simulink model "TP_4"  (R2022a)
settings: Solver=VariableStepAuto  StartTime=0.0  StopTime=10.0  RelTol=1e-3
undefined symbols (not defined in the file): g, l
settings Model: Creator=acanon  LastModifiedBy=acanon

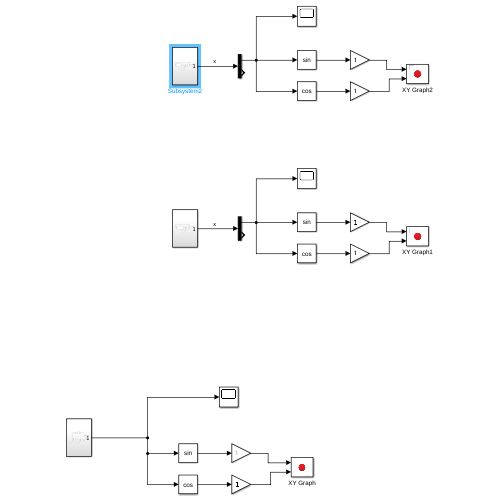
[thumbnail: Simulink's stored preview of the top-level diagram]
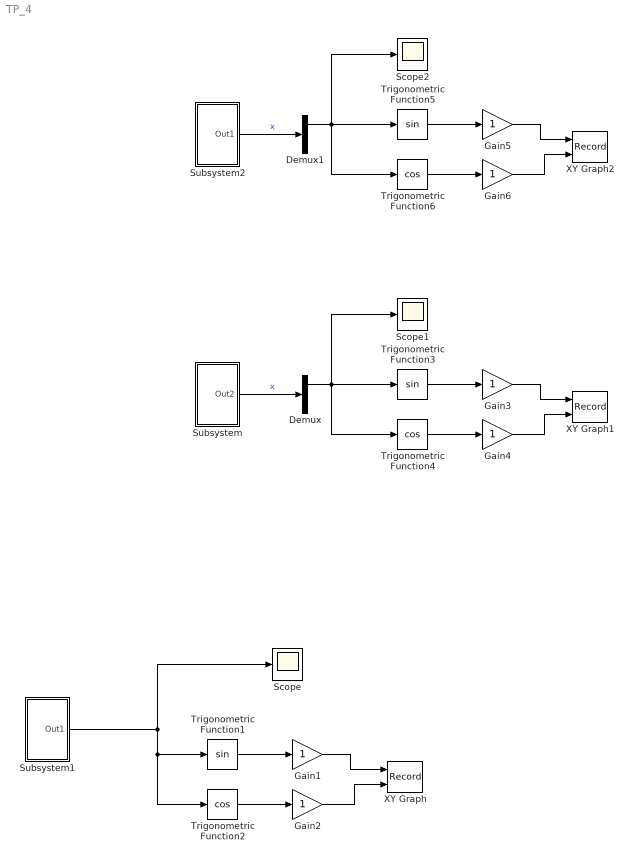
== system TP_4 ==
  Demux : Demux  Outputs=2
  Demux1 : Demux  Outputs=2
  Gain{1..6} (6 alike) : Gain
  Scope : Scope
  Scope1 : Scope
  Scope2 : Scope
  Subsystem : Subsystem
  Subsystem1 : Subsystem
  Subsystem2 : Subsystem
  Trigonometric Function1 : Trigonometry
  Trigonometric Function2 : Trigonometry  Operator=cos
  Trigonometric Function3 : Trigonometry
  Trigonometric Function4 : Trigonometry  Operator=cos
  Trigonometric Function5 : Trigonometry
  Trigonometric Function6 : Trigonometry  Operator=cos
  XY Graph : Record  FileSettingsInternal="{\"entries\":[{\"content\":{\"excelSettings\":{\"content\":{},\"type\":\"Streamout.ExcelSettings\"}},\"type\":\"Streamout.FileSettingStorage\",\"uuid\":\"6b5f49a7-b3b1-4d7e-bc90-530d4034afb4\"}],\"packageUris\":[\"http://schema.mathworks.com/mf0/streamout_blocks/R2020a\"],\"version\":\"1.0\"}"  Layout=[1 1]  SignalsInternal="{\"entries\":[{\"content\":{\"signals\":[{\"content\":{\"blockPath\":[\"TP_4/XY Graph\"],\"channel\":[],\"dimensions\":[1],\"domain\":\"TP_4/XY Graph\",\"lineColor\":\"#a2142f\",\"plots\":[1],\"port\":1,\"sid\":[\"\"],\"signalID\":770,\"signalName\":\"Gain1\"},\"type\":\"RecordBlkView.Signal\",\"uuid\":\"252f4a16-2fdb-4508-836e-7d7f95c59b1a\"},{\"content\":{\"blockPath\":[\"TP_4/XY Graph\"],\"channel\":[],\"dimensions\":[1],\"domain\":\"TP_4/XY Graph\",\"lineColor\":\"#139fff\",\"plots\":[1],\"port\":2,\"sid\":[\"\"],\"signalID\":774,\"signalName\":\"Gain2\"},\"type\":\"RecordBlkView.Signal\",\"uuid\":\"1550168d-e5f5-498f-8827-b1f3ffe8fbd9\"}]},\"type\":\"RecordBlkView.InputSignals\",\"uuid\":\"ba0f4b2c-9202-4a03-ae75-802def453182\"}],\"packageUris\":[\"http://schema.mathworks.com/mf0/streamout_blocks/R2020a\"],\"version\":\"1.0\"}"  VisualizationBindings="{\"xyplotplugin\":{\"info\":[{\"series\":[{\"bindingParametersList\":[{\"parameter\":\"X-Axis\",\"signalID\":770,\"signalName\":\"Gain1\"},{\"parameter\":\"Y-Axis\",\"signalID\":774,\"signalName\":\"Gain2\"}],\"seriesID\":7779}],\"subplotID\":1}]}}"  CompatibilityTag=XY
  XY Graph1 : Record  FileSettingsInternal="{\"entries\":[{\"content\":{\"excelSettings\":{\"content\":{},\"type\":\"Streamout.ExcelSettings\"}},\"type\":\"Streamout.FileSettingStorage\",\"uuid\":\"647a4500-99ce-4aa8-8361-fcd857458ba3\"}],\"packageUris\":[\"http://schema.mathworks.com/mf0/streamout_blocks/R2020a\"],\"version\":\"1.0\"}"  Layout=[1 1]  SignalsInternal="{\"entries\":[{\"content\":{\"signals\":[{\"content\":{\"blockPath\":[\"TP_4/XY Graph1\"],\"channel\":[],\"dimensions\":[1],\"domain\":\"TP_4/XY Graph1\",\"lineColor\":\"#a2142f\",\"plots\":[1],\"port\":1,\"sid\":[\"\"],\"signalID\":754,\"signalName\":\"Gain3\"},\"type\":\"RecordBlkView.Signal\",\"uuid\":\"8e395301-b303-424e-a96f-b943253f827c\"},{\"content\":{\"blockPath\":[\"TP_4/XY Graph1\"],\"channel\":[],\"dimensions\":[1],\"domain\":\"TP_4/XY Graph1\",\"lineColor\":\"#139fff\",\"plots\":[1],\"port\":2,\"sid\":[\"\"],\"signalID\":758,\"signalName\":\"Gain4\"},\"type\":\"RecordBlkView.Signal\",\"uuid\":\"861f5d7e-9fe7-4d07-8f40-ba319954fb9d\"}]},\"type\":\"RecordBlkView.InputSignals\",\"uuid\":\"dfbe973e-b0a0-4eca-b465-339f94536037\"}],\"packageUris\":[\"http://schema.mathworks.com/mf0/streamout_blocks/R2020a\"],\"version\":\"1.0\"}"  VisualizationBindings="{\"xyplotplugin\":{\"info\":[{\"series\":[{\"bindingParametersList\":[{\"parameter\":\"X-Axis\",\"signalID\":754,\"signalName\":\"Gain3\"},{\"parameter\":\"Y-Axis\",\"signalID\":758,\"signalName\":\"Gain4\"}],\"seriesID\":52056}],\"subplotID\":1}]}}"  CompatibilityTag=XY
  XY Graph2 : Record  FileSettingsInternal="{\"entries\":[{\"content\":{\"excelSettings\":{\"content\":{},\"type\":\"Streamout.ExcelSettings\"}},\"type\":\"Streamout.FileSettingStorage\",\"uuid\":\"91d296fc-894f-4125-a729-7558be06892a\"}],\"packageUris\":[\"http://schema.mathworks.com/mf0/streamout_blocks/R2020a\"],\"version\":\"1.0\"}"  Layout=[1 1]  SignalsInternal="{\"entries\":[{\"content\":{\"signals\":[{\"content\":{\"blockPath\":[\"TP_4/XY Graph2\"],\"channel\":[],\"dimensions\":[1,1],\"domain\":\"TP_4/XY Graph2\",\"lineColor\":\"#a2142f\",\"plots\":[1],\"port\":1,\"sid\":[\"\"],\"signalID\":762,\"signalName\":\"Gain5\"},\"type\":\"RecordBlkView.Signal\",\"uuid\":\"373c4582-ecbd-4420-a1ec-272adeca90e9\"},{\"content\":{\"blockPath\":[\"TP_4/XY Graph2\"],\"channel\":[],\"dimensions\":[1,1],\"domain\":\"TP_4/XY Graph2\",\"lineColor\":\"#139fff\",\"plots\":[1],\"port\":2,\"sid\":[\"\"],\"signalID\":766,\"signalName\":\"Gain6\"},\"type\":\"RecordBlkView.Signal\",\"uuid\":\"e2adde95-3a69-431b-804e-fdc9e32eb17f\"}]},\"type\":\"RecordBlkView.InputSignals\",\"uuid\":\"6b5ed82e-5b03-46e4-8a06-dd9cee375b8d\"}],\"packageUris\":[\"http://schema.mathworks.com/mf0/streamout_blocks/R2020a\"],\"version\":\"1.0\"}"  VisualizationBindings="{\"xyplotplugin\":{\"info\":[{\"series\":[{\"bindingParametersList\":[{\"parameter\":\"X-Axis\",\"signalID\":762,\"signalName\":\"Gain5\"},{\"parameter\":\"Y-Axis\",\"signalID\":766,\"signalName\":\"Gain6\"}],\"seriesID\":34063}],\"subplotID\":1}]}}"  CompatibilityTag=XY
  wires:
  Trigonometric Function1/1 -> Gain1/1
  Trigonometric Function2/1 -> Gain2/1
  Gain1/1 -> XY Graph/1
  Gain2/1 -> XY Graph/2
  Subsystem1/1(Out1) -> Trigonometric Function2/1, Trigonometric Function1/1, Scope/1
  Demux/1 -> Scope1/1, Trigonometric Function3/1, Trigonometric Function4/1
  Gain4/1 -> XY Graph1/2
  Gain3/1 -> XY Graph1/1
  Trigonometric Function4/1 -> Gain4/1
  Trigonometric Function3/1 -> Gain3/1
  Subsystem/1(Out2) -> Demux/1  "x"
  Subsystem2/1(Out1) -> Demux1/1  "x"
  Trigonometric Function5/1 -> Gain5/1
  Trigonometric Function6/1 -> Gain6/1
  Gain5/1 -> XY Graph2/1
  Gain6/1 -> XY Graph2/2
  Demux1/1 -> Trigonometric Function6/1, Trigonometric Function5/1, Scope2/1

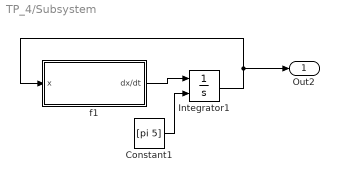
== system TP_4/Subsystem ==
  Constant1 : Constant  Value=[pi 5]
  Integrator1 : Integrator  InitialConditionSource=external
  f1 : Subsystem
  Out2 : Outport
  wires:
  Integrator1/1 -> f1/1(x), Out2/1
  Constant1/1 -> Integrator1/2
  f1/1(dx/dt) -> Integrator1/1

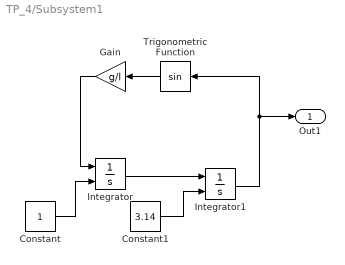
== system TP_4/Subsystem1 ==
  Constant : Constant
  Constant1 : Constant  Value=3.14
  Gain : Gain  Gain=g/l
  Integrator : Integrator  InitialConditionSource=external
  Integrator1 : Integrator  InitialConditionSource=external
  Trigonometric Function : Trigonometry
  Out1 : Outport
  wires:
  Integrator/1 -> Integrator1/1
  Constant1/1 -> Integrator1/2
  Trigonometric Function/1 -> Gain/1
  Gain/1 -> Integrator/1
  Integrator1/1 -> Trigonometric Function/1, Out1/1
  Constant/1 -> Integrator/2

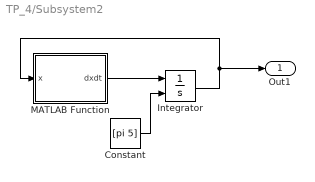
== system TP_4/Subsystem2 ==
  Constant : Constant  Value=[pi 5]
  Integrator : Integrator  InitialConditionSource=external
  MATLAB Function : MATLAB Function  TreatAsAtomicUnit=on
  Out1 : Outport
  wires:
  Constant/1 -> Integrator/2
  MATLAB Function/1(dxdt) -> Integrator/1
  Integrator/1 -> MATLAB Function/1(x), Out1/1

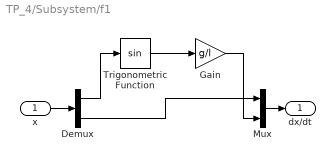
== system TP_4/Subsystem/f1 ==
  x : Inport
  Demux : Demux  Outputs=2
  Gain : Gain  Gain=g/l
  Mux : Mux  Inputs=2
  Trigonometric Function : Trigonometry
  dx/dt : Outport
  wires:
  Gain/1 -> Mux/2
  Trigonometric Function/1 -> Gain/1
  Demux/1 -> Trigonometric Function/1
  Demux/2 -> Mux/1
  Mux/1 -> dx/dt/1
  x/1 -> Demux/1

== matlab function TP_4/Subsystem2/MATLAB Function ==
  data: x input; dxdt output
function dxdt = fcn(x)
    dxdt = [x(2) sin(x(1))*9.81/1];
